simulink model "Control2"  (R2020b)
settings: Solver=FixedStepAuto  StartTime=0.0  StopTime=100.0  FixedStep=0.01  RelTol=1e-3
libraries: PB_Library_Master x2, simulink x1, Lib_Solve_SSNRSolverJC_TMATS x1
settings Model: Creator=gfretti  LastModifiedBy=nbutler2
settings SFSimCC: CustomCodeUndefinedFunction=UseInterfaceOnly

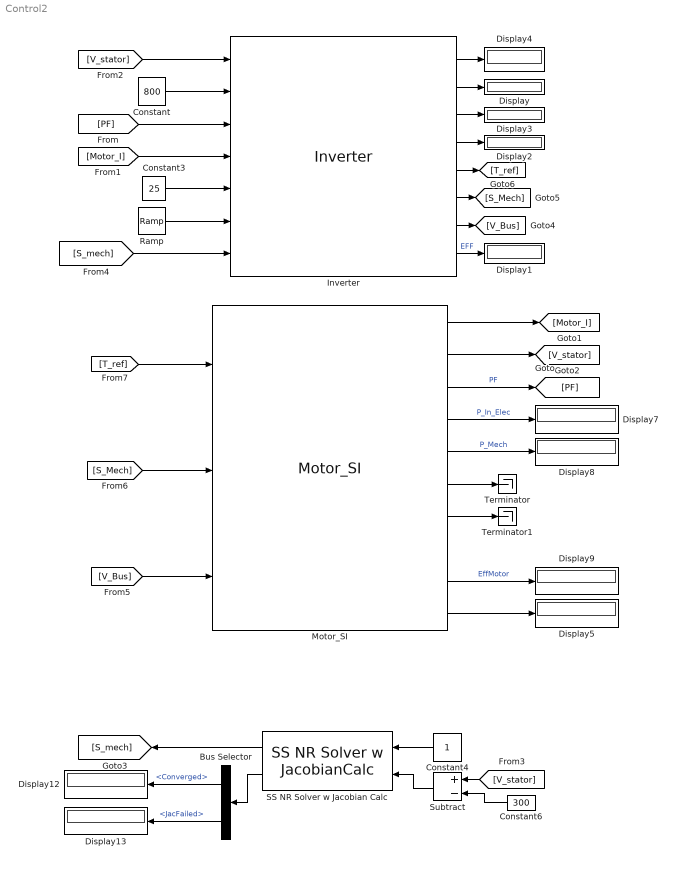
== system Control2 ==
  Bus Selector : BusSelector  OutputSignals=Converged,JacFailed
  Constant : Constant  Value=800
  Constant3 : Constant  Value=25
  Constant4 : Constant
  Constant6 : Constant  Value=300
  Display{,1..5,7..9,12..13} (11 alike) : Display
  Inverter : PB_Library_Master/Inverter  T_M=[25 175]  u_D_M=[1.16666666666667 0.999999999999998]  u_ce0_M=[0.971428571428571 0.848275862068965]  R_c_M=[0.0285714285714286 0.0551724137931034]  R_D_M=[0.0238095238095238 0.0294117647058824]  E0_M=[6.00000000000002e-05 6.00000000000002e-05]  E1_M=[5.6e-05 5.6e-05]  f_sw_M=20000  L_s_M=0.00115  P_max_I=22000  V_phase_I=400  f_sw_I=0  L_s_I=.00086+0.00029
  Motor_SI : PB_Library_Master/Motor_SI  pp=2  flux_m=0.57773  R_s=0.032  L_s=0.00115  P_Fe_Nom=904.3614  S_nom=3000  T_nom=70  P_out_max=22000  I_max=36.5  P_in_max=30000  T_max=80  MassEst_M=136.5892  Poles_i=4  R_s_i=.032  L_s_i=.00086+0.00029  S_nom_i=3000  T_nom_i=70  P_out_max_i=22000  I_max_i=36.5  P_in_max_i=30000  K_i=121  V_nom_i=368  T_max_i=80  CalculatePFe=Compute iron losses automatically  P_Fe_Nom_i=0  I_nom_i=36.5  PF_nom_i=0.99  P_Fe_Calc_Flag=1
  Ramp : simulink/Sources/Ramp  slope=-1  start=0  InitialOutput=50
  SS NR Solver w Jacobian Calc : Lib_Solve_SSNRSolverJC_TMATS/SS NR Solver w JacobianCalc  SJac_Per_M=[-0.1;-0.01;0.01;0.1]  SNR_IC_M=2450  SNR_DX_M=100  SNR_Mx_M=100000  SNR_Mn_M=-100000  SJacobianAttempts_M=2*10^5  Cond_Limits_M=0.01
  Subtract : Sum  Inputs=+-
  Terminator : Terminator
  Terminator1 : Terminator
  wires:
  Inverter/5 -> [T_ref]
  Inverter/6 -> [S_Mech]
  Inverter/7 -> [V_Bus]
  Motor_SI/2 -> [V_stator]
  Motor_SI/3 -> [PF]  "PF"
  Constant/1 -> Inverter/2
  Inverter/2 -> Display/1
  Inverter/8 -> Display1/1  "EFF"
  Inverter/4 -> Display2/1
  Inverter/3 -> Display3/1
  Inverter/1 -> Display4/1
  Motor_SI/10 -> Display5/1
  Constant3/1 -> Inverter/5
  Motor_SI/1 -> [Motor_I]
  Bus Selector/1 -> Display12/1  "<Converged>"
  Bus Selector/2 -> Display13/1  "<JacFailed>"
  SS NR Solver w Jacobian Calc/2 -> Bus Selector/1
  Constant4/1 -> SS NR Solver w Jacobian Calc/1
  Subtract/1 -> SS NR Solver w Jacobian Calc/2
  Constant6/1 -> Subtract/2
  Ramp/1 -> Inverter/6
  SS NR Solver w Jacobian Calc/1 -> [S_mech]
  Motor_SI/4 -> Display7/1  "P_In_Elec"
  Motor_SI/5 -> Display8/1  "P_Mech"
  Motor_SI/9 -> Display9/1  "EffMotor"
  Motor_SI/6 -> Terminator/1
  Motor_SI/7 -> Terminator1/1
  [PF] -> Inverter/3
  [Motor_I] -> Inverter/4
  [V_stator] -> Inverter/1
  [V_stator] -> Subtract/1
  [S_mech] -> Inverter/7
  [V_Bus] -> Motor_SI/3
  [S_Mech] -> Motor_SI/2
  [T_ref] -> Motor_SI/1
